simulink library "dpsba_custom"  (R2018b)
settings: Solver=VariableStepAuto  StartTime=0.0  StopTime=10.0  RelTol=1e-3
undefined symbols (not defined in the file or in its folder): AdvDSPBChannelOutDisplay, AStInput, AStOutput, dspba_ChannelInVis, dspba_ChannelOutVis, dspba_internal_get_channel_ports, DSPBAAvalonST, latency
libraries: DSPBAPrim x6
settings Model: Creator=trevorvannoy  LastModifiedBy=trevorvannoy

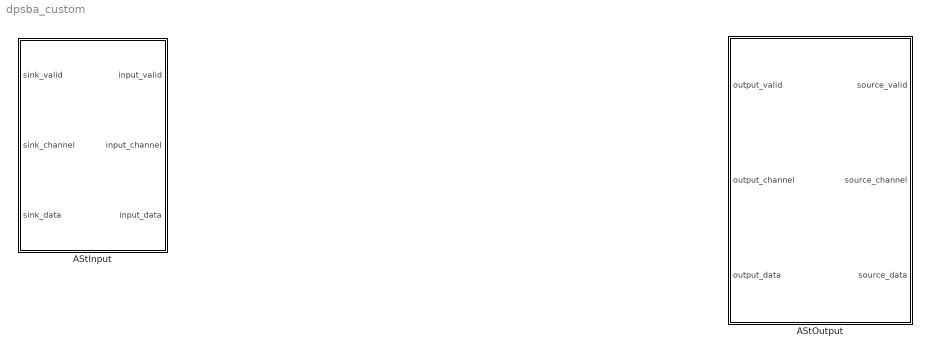
== system dpsba_custom ==
  AStInput : Subsystem  AncestorBlock=DSPBAAvalonST/AStInput  InitFcn=warning('off','Simulink:Commands:LoadMdlParameterizedLink');  StopFcn=warning('on','Simulink:Commands:LoadMdlParameterizedLink');  mask(DSP Builder Advanced Blockset Avalon Streaming Input Interface){}
      mask help:
      | Avalon Streaming Input Interface
      |
      | Place this block at the front end of a system to generate the appropriate hw.tcl code for an Avalon Streaming interface with same name as the name of this block.
      mask Help: helpview(dspba.GetHelp('AStInput'));
      mask Display:
      | image('dspba_channel.jpg');
      | fprintf('Avalon-ST\nInput');
      | port_label('input',1,'sink_valid');
      | port_label('input',2,'sink_channel');
      | port_label('input',3,'sink_data');
      | port_label('output',1,'input_valid');
      | port_label('output',2,'input_channel');
      | port_label('output',3,'input_data');
  AStOutput : Subsystem  AncestorBlock=DSPBAAvalonST/AStOutput  InitFcn=warning('off','Simulink:Commands:LoadMdlParameterizedLink');  StopFcn=warning('on','Simulink:Commands:LoadMdlParameterizedLink');  mask(DSP Builder Advanced Blockset Avalon Streaming Output Interface){fifo_setup=[32 1 20]}
      mask prompts: fifo_setup "FIFO Setup [<_depth> <_fill_threshold> <_full_period>]:"
      mask help:
      | Avalon Streaming Output Interface
      |
      | Place this block the back end of a system to generate the appropriate hw.tcl code for an Avalon Streaming interface with same name as the name of this block.
      mask Help: helpview(dspba.GetHelp('AStOutput'));
      mask Display:
      | image('dspba_channel.jpg');
      | fprintf('Avalon-ST\nOutput');
      | port_label('input',1,'output_valid');
      | port_label('input',2,'output_channel');
      | port_label('input',3,'output_data');
      | port_label('output',1,'source_valid');
      | port_label('output',2,'source_channel');
      | port_label('output',3,'source_data');

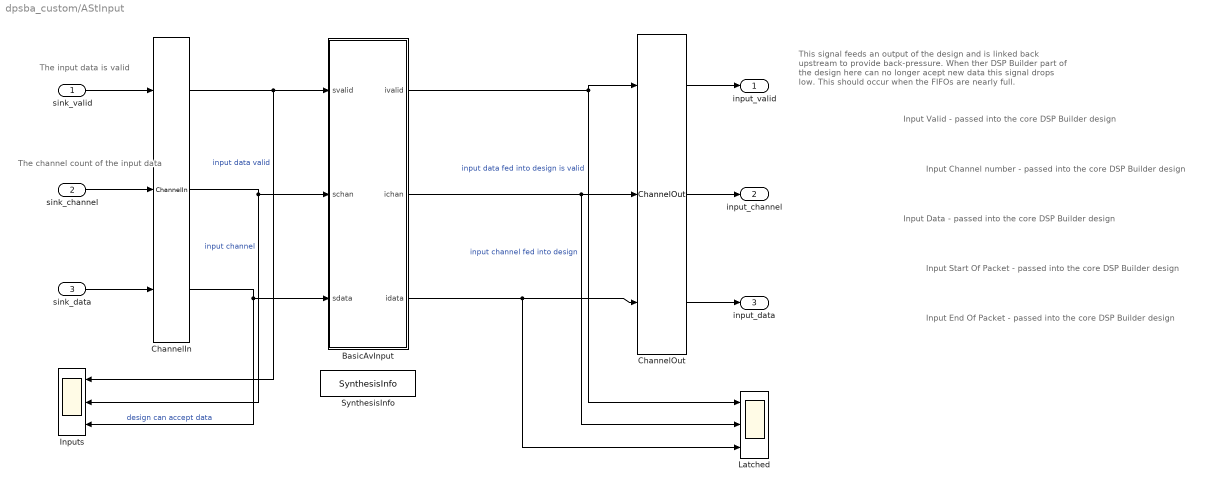
== system dpsba_custom/AStInput ==
  note: Input End Of Packet - passed into the core DSP Builder design
  note: Input Start Of Packet - passed into the core DSP Builder design
  note: Input Data - passed into the core DSP Builder design
  note: Input Valid - passed into the core DSP Builder design
  note: This signal feeds an output of the design and is linked back
      | upstream to provide back-pressure. When ther DSP Builder
      | part of the design here can no longer acept new data this
      | signal drops low. This should occur when the FIFOs are nearly
      | full.
  note: Input Channel number - passed into the core DSP Builder design
  note: The channel count of the input data
  note: The input data is valid
  sink_valid : Inport  Tag=valid
      settings: AttributesFormatString=%<Tag>
  sink_channel : Inport  Tag=channel  Port=2
      settings: AttributesFormatString=%<Tag>
  sink_data : Inport  Tag=data  Port=3
      settings: AttributesFormatString=%<Tag>
  BasicAvInput : Subsystem
  ChannelIn : DSPBAPrim/ChannelIn  primtype=channelin  nInputs=dspba_internal_get_channel_ports(gcb)  nOutputs=dspba_internal_get_channel_ports(gcb)  omode=Inherit via internal rule  otype=sfix(16)  scale=2^-15  rndmethod=Unbiased  factor=1  satmethod=Symmetric  shift_vec=[0 1 2 -1]  value=1  inPortNames=['v'; 'c'; '0'; '1'; '2'; '3'; '4'; '5'; '6'; '7'; '8'; '9'; 'A'; 'B'; 'D'; 'E'; 'F'; 'G'; 'H'; 'I'; 'J'; 'K'; 'L'; 'M'; 'N'; 'O'; 'P'; 'Q'; 'R'; 'S'; 'T'; 'U'; 'W'; 'X'; 'Y'; 'Z']  outPortNames=['v'; 'c'; '0'; '1'; '2'; '3'; '4'; '5'; '6'; '7'; '8'; '9'; 'A'; 'B'; 'D'; 'E'; 'F'; 'G'; 'H'; 'I'; 'J'; 'K'; 'L'; 'M'; 'N'; 'O'; 'P'; 'Q'; 'R'; 'S'; 'T'; 'U'; 'W'; 'X'; 'Y'; 'Z']  dspbaimage=dspba_prim.jpg  text=fprintf('In');  style=Optimised  dataSignals=1  foldingEnabled=off  channels=1  sampleRate=200  packetBeginPresent=off  packetBeginEnabled=off  visibilities=dspba_ChannelInVis(gcb)  latencyCorrection=0  scheduleOrigin=on  version=20141013
  ChannelOut : DSPBAPrim/ChannelOut  primtype=channelout  nInputs=dspba_internal_get_channel_ports(gcb)  nOutputs=dspba_internal_get_channel_ports(gcb)  omode=Inherit via internal rule  otype=sfix(16)  scale=2^-15  rndmethod=Unbiased  factor=1  satmethod=Symmetric  shift_vec=[0 1 2 -1]  value=1  inPortNames=['v'; 'c'; '0'; '1'; '2'; '3'; '4'; '5'; '6'; '7'; '8'; '9'; 'A'; 'B'; 'D'; 'E'; 'F'; 'G'; 'H'; 'I'; 'J'; 'K'; 'L'; 'M'; 'N'; 'O'; 'P'; 'Q'; 'R'; 'S'; 'T'; 'U'; 'W'; 'X'; 'Y'; 'Z']  outPortNames=['v'; 'c'; '0'; '1'; '2'; '3'; '4'; '5'; '6'; '7'; '8'; '9'; 'A'; 'B'; 'D'; 'E'; 'F'; 'G'; 'H'; 'I'; 'J'; 'K'; 'L'; 'M'; 'N'; 'O'; 'P'; 'Q'; 'R'; 'S'; 'T'; 'U'; 'W'; 'X'; 'Y'; 'Z']  dspbaimage=dspba_prim.jpg  text=fprintf('Out%s', AdvDSPBChannelOutDisplay(latency));  style=Optimised  dataSignals=1  foldingEnabled=off  channels=1  sampleRate=200  packetBeginPresent=off  packetBeginEnabled=off  visibilities=dspba_ChannelOutVis(gcb)  latency=0  latencyCorrection=0  version=20141013
  Inputs : Scope  NumInputPorts=3
  Latched : Scope  NumInputPorts=3
  SynthesisInfo : DSPBAPrim/SynthesisInfo  primtype=synthinfo  nInputs=0  nOutputs=0  omode=Inherit via internal rule  otype=sfix(16)  scale=2^-15  rndmethod=Truncate  factor=1  satmethod=Symmetric  shift_vec=[0 1 2 -1]  value=99  inPortNames=[' '; ' ';]  outPortNames=[' ']  dspbaimage=dspba_prim_ctrl.jpg  text=fprintf('Style=%s', style);  style=Scheduled  visibilities=32768  constraintInUse=on  constraintRelation==  constraintLimit=0  bitAccurate=off  version=20150220
  input_valid : Outport  Tag=valid
      settings: AttributesFormatString=%<Tag>
  input_channel : Outport  Tag=channel  Port=2
      settings: AttributesFormatString=%<Tag>
  input_data : Outport  Tag=data  Port=3
      settings: AttributesFormatString=%<Tag>
  wires:
  ChannelOut/3 -> input_data/1
  BasicAvInput/1(ivalid) -> Latched/1, ChannelOut/1  "input data fed into design is valid"
  BasicAvInput/2(ichan) -> ChannelOut/2, Latched/2  "input channel fed into design"
  BasicAvInput/3(idata) -> Latched/3, ChannelOut/3
  ChannelIn/1 -> Inputs/1, BasicAvInput/1(svalid)  "input data valid"
  ChannelIn/2 -> Inputs/2, BasicAvInput/2(schan)  "input channel"
  ChannelIn/3 -> BasicAvInput/3(sdata), Inputs/3  "design can accept data"
  sink_valid/1 -> ChannelIn/1
  sink_channel/1 -> ChannelIn/2
  sink_data/1 -> ChannelIn/3
  ChannelOut/1 -> input_valid/1
  ChannelOut/2 -> input_channel/1

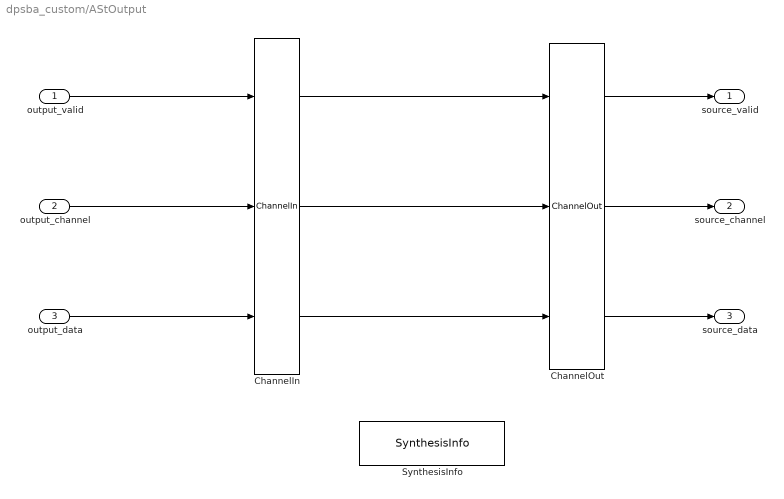
== system dpsba_custom/AStOutput ==
  output_valid : Inport  Tag=valid
      settings: AttributesFormatString=%<Tag>
  output_channel : Inport  Tag=channel  Port=2
      settings: AttributesFormatString=%<Tag>
  output_data : Inport  Tag=data  Port=3
      settings: AttributesFormatString=%<Tag>
  ChannelIn : DSPBAPrim/ChannelIn  primtype=channelin  nInputs=dspba_internal_get_channel_ports(gcb)  nOutputs=dspba_internal_get_channel_ports(gcb)  omode=Inherit via internal rule  otype=sfix(16)  scale=2^-15  rndmethod=Unbiased  factor=1  satmethod=Symmetric  shift_vec=[0 1 2 -1]  value=1  inPortNames=['v'; 'c'; '0'; '1'; '2'; '3'; '4'; '5'; '6'; '7'; '8'; '9'; 'A'; 'B'; 'D'; 'E'; 'F'; 'G'; 'H'; 'I'; 'J'; 'K'; 'L'; 'M'; 'N'; 'O'; 'P'; 'Q'; 'R'; 'S'; 'T'; 'U'; 'W'; 'X'; 'Y'; 'Z']  outPortNames=['v'; 'c'; '0'; '1'; '2'; '3'; '4'; '5'; '6'; '7'; '8'; '9'; 'A'; 'B'; 'D'; 'E'; 'F'; 'G'; 'H'; 'I'; 'J'; 'K'; 'L'; 'M'; 'N'; 'O'; 'P'; 'Q'; 'R'; 'S'; 'T'; 'U'; 'W'; 'X'; 'Y'; 'Z']  dspbaimage=dspba_prim.jpg  text=fprintf('In');  style=Optimised  dataSignals=1  foldingEnabled=off  channels=1  sampleRate=200  packetBeginPresent=off  packetBeginEnabled=off  visibilities=dspba_ChannelInVis(gcb)  latencyCorrection=0  scheduleOrigin=on  version=20141013
  ChannelOut : DSPBAPrim/ChannelOut  primtype=channelout  nInputs=dspba_internal_get_channel_ports(gcb)  nOutputs=dspba_internal_get_channel_ports(gcb)  omode=Inherit via internal rule  otype=sfix(16)  scale=2^-15  rndmethod=Unbiased  factor=1  satmethod=Symmetric  shift_vec=[0 1 2 -1]  value=1  inPortNames=['v'; 'c'; '0'; '1'; '2'; '3'; '4'; '5'; '6'; '7'; '8'; '9'; 'A'; 'B'; 'D'; 'E'; 'F'; 'G'; 'H'; 'I'; 'J'; 'K'; 'L'; 'M'; 'N'; 'O'; 'P'; 'Q'; 'R'; 'S'; 'T'; 'U'; 'W'; 'X'; 'Y'; 'Z']  outPortNames=['v'; 'c'; '0'; '1'; '2'; '3'; '4'; '5'; '6'; '7'; '8'; '9'; 'A'; 'B'; 'D'; 'E'; 'F'; 'G'; 'H'; 'I'; 'J'; 'K'; 'L'; 'M'; 'N'; 'O'; 'P'; 'Q'; 'R'; 'S'; 'T'; 'U'; 'W'; 'X'; 'Y'; 'Z']  dspbaimage=dspba_prim.jpg  text=fprintf('Out%s', AdvDSPBChannelOutDisplay(latency));  style=Optimised  dataSignals=1  foldingEnabled=off  channels=1  sampleRate=200  packetBeginPresent=off  packetBeginEnabled=off  visibilities=dspba_ChannelOutVis(gcb)  latency=0  latencyCorrection=0  version=20141013
  SynthesisInfo : DSPBAPrim/SynthesisInfo  primtype=synthinfo  nInputs=0  nOutputs=0  omode=Inherit via internal rule  otype=sfix(16)  scale=2^-15  rndmethod=Truncate  factor=1  satmethod=Symmetric  shift_vec=[0 1 2 -1]  value=99  inPortNames=[' '; ' ';]  outPortNames=[' ']  dspbaimage=dspba_prim_ctrl.jpg  text=fprintf('Style=%s', style);  style=Scheduled  visibilities=32768  constraintInUse=on  constraintRelation==  constraintLimit=0  bitAccurate=off  version=20150220
  source_valid : Outport  Tag=valid
      settings: AttributesFormatString=%<Tag>
  source_channel : Outport  Tag=channel  Port=2
      settings: AttributesFormatString=%<Tag>
  source_data : Outport  Tag=data  Port=3
      settings: AttributesFormatString=%<Tag>
  wires:
  output_valid/1 -> ChannelIn/1
  output_channel/1 -> ChannelIn/2
  output_data/1 -> ChannelIn/3
  ChannelOut/1 -> source_valid/1
  ChannelOut/2 -> source_channel/1
  ChannelOut/3 -> source_data/1
  ChannelIn/1 -> ChannelOut/1
  ChannelIn/2 -> ChannelOut/2
  ChannelIn/3 -> ChannelOut/3

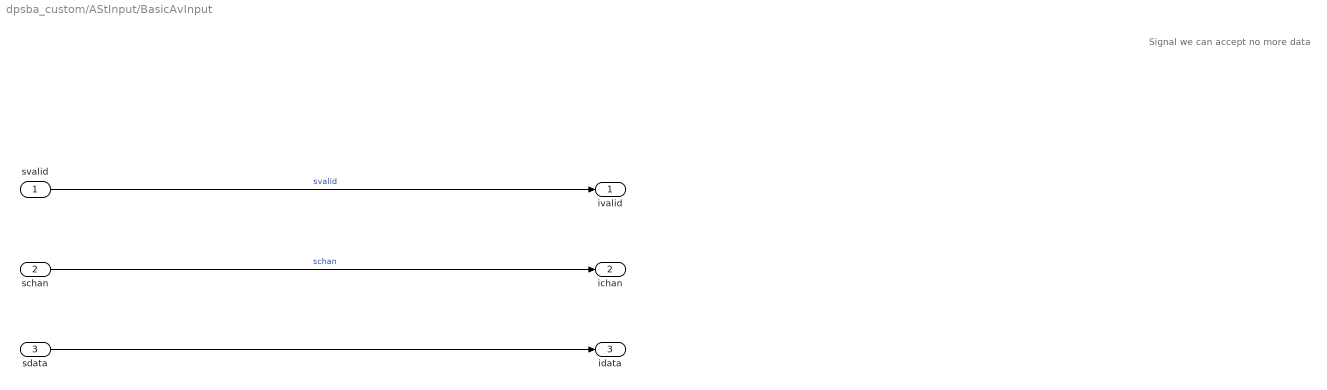
== system dpsba_custom/AStInput/BasicAvInput ==
  note: Signal we can accept no more data
  svalid : Inport
  schan : Inport  Port=2
  sdata : Inport  Port=3
  ivalid : Outport
  ichan : Outport  Port=2
  idata : Outport  Port=3
  wires:
  svalid/1 -> ivalid/1  "svalid"
  sdata/1 -> idata/1
  schan/1 -> ichan/1  "schan"
